simulink model "adaptive_control"  (R2020b)
settings: Solver=VariableStepAuto  StartTime=0.0  StopTime=30  RelTol=1e-3
values from neighbouring files (symbols this model uses):
  A = 1    [hw8_main.m]
  ddq_d = 0    [hw8_main.m]
  dq_d = 0    [hw8_main.m]
  F_hat0 = oneDof.F*0.8    [hw8_main.m]
  Fc = 1    [hw8_main.m]
  G_hat0 = oneDof.G*0.8    [hw8_main.m]
  I_hat0 = oneDof.I*0.8    [hw8_main.m]
  K_D = 100    [hw8_main.m]
  K_theta_inv = inv(K_theta)    [hw8_main.m]
  Lamba = 50    [hw8_main.m]
undefined symbols (not defined in the file or in its folder): oneDof
settings Model: Creator=nicol  LastModifiedBy=nicol

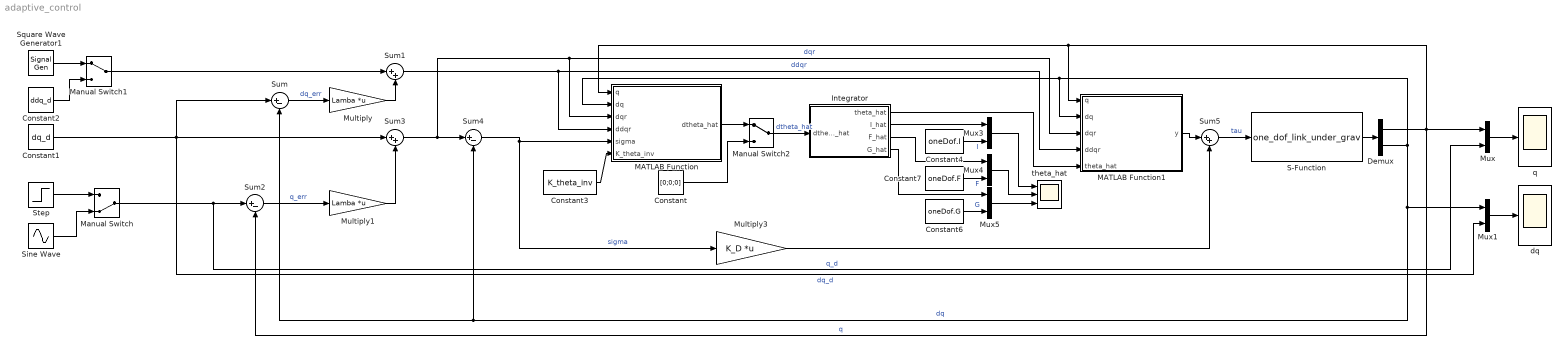
== system adaptive_control ==
  Constant : Constant  Value=[0;0;0]
  Constant1 : Constant  Value=dq_d
  Constant2 : Constant  Value=ddq_d
  Constant3 : Constant  Value=K_theta_inv
  Constant4 : Constant  Value=oneDof.I
  Constant6 : Constant  Value=oneDof.G
  Constant7 : Constant  Value=oneDof.F
  Demux : Demux  Outputs=2
  Integrator : Subsystem
  MATLAB Function : MATLAB Function  TreatAsAtomicUnit=on
  MATLAB Function1 : MATLAB Function  TreatAsAtomicUnit=on
  Manual Switch : ManualSwitch  CurrentSetting=0
  Manual Switch1 : ManualSwitch
  Manual Switch2 : ManualSwitch
  Multiply : Gain  Gain=Lamba  Multiplication=Matrix(K*u)
  Multiply1 : Gain  Gain=Lamba  Multiplication=Matrix(K*u)
  Multiply3 : Gain  Gain=K_D  Multiplication=Matrix(K*u)
  Mux{,1,3..5} (5 alike) : Mux  Inputs=2
  S-Function : S-Function  FunctionName=one_dof_link_under_grav  Parameters=oneDof  SFunctionDeploymentMode=off  EnableBusSupport=off
  Sine Wave : Sin  Amplitude=A  Frequency=Fc  SampleTime=0
  Square Wave Generator1 : SignalGenerator  WaveForm=square  Amplitude=A  Units=rad/sec
  Step : Step  After=A  SampleTime=0
  Sum : Sum  Inputs=|+-
  Sum1 : Sum  Inputs=|++
  Sum2 : Sum  Inputs=|+-
  Sum3 : Sum  Inputs=|++
  Sum4 : Sum  Inputs=|+-
  Sum5 : Sum  Inputs=|++
  dq : Scope
  q : Scope
  theta_hat : Scope  NumInputPorts=3
  wires:
  Sum/1 -> Multiply/1  "dq_err"
  Constant1/1 -> Mux1/2, Sum3/1, Sum/1  "dq_d"
  Manual Switch1/1 -> Sum1/1
  Multiply/1 -> Sum1/2
  Manual Switch/1 -> Mux/2, Sum2/1  "q_d"
  Sum2/1 -> Multiply1/1  "q_err"
  Sum3/1 -> Sum4/1, MATLAB Function/3(dqr), MATLAB Function1/3(dqr)  "dqr"
  Multiply1/1 -> Sum3/2
  Sum4/1 -> MATLAB Function/5(sigma), Multiply3/1  "sigma"
  MATLAB Function/1(dtheta_hat) -> Manual Switch2/1
  MATLAB Function1/1(y) -> Sum5/1
  Multiply3/1 -> Sum5/2
  Demux/1 -> MATLAB Function1/1(q), MATLAB Function/1(q), Mux/1, Sum2/2  "q"
  S-Function/1 -> Demux/1
  Sum5/1 -> S-Function/1  "tau"
  Demux/2 -> MATLAB Function1/2(dq), MATLAB Function/2(dq), Mux1/1, Sum4/2, Sum/2  "dq"
  Sum1/1 -> MATLAB Function/4(ddqr), MATLAB Function1/4(ddqr)  "ddqr"
  Mux1/1 -> dq/1
  Mux/1 -> q/1
  Constant3/1 -> MATLAB Function/6(K_theta_inv)
  Sine Wave/1 -> Manual Switch/2
  Square Wave Generator1/1 -> Manual Switch1/1
  Constant2/1 -> Manual Switch1/2
  Step/1 -> Manual Switch/1
  Constant/1 -> Manual Switch2/2
  Constant4/1 -> Mux3/2  "I"
  Mux4/1 -> theta_hat/2
  Constant7/1 -> Mux4/2  "F"
  Constant6/1 -> Mux5/2  "G"
  Mux5/1 -> theta_hat/3
  Mux3/1 -> theta_hat/1
  Manual Switch2/1 -> Integrator/1(dtheta_hat)  "dtheta_hat"
  Integrator/2(I_hat) -> Mux3/1
  Integrator/1(theta_hat) -> MATLAB Function1/5(theta_hat)
  Integrator/3(F_hat) -> Mux4/1
  Integrator/4(G_hat) -> Mux5/1

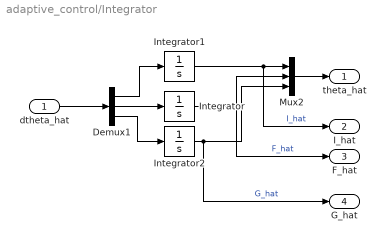
== system adaptive_control/Integrator ==
  dtheta_hat : Inport
  Demux1 : Demux  Outputs=3
  Integrator : Integrator  InitialCondition=F_hat0
  Integrator1 : Integrator  InitialCondition=I_hat0
  Integrator2 : Integrator  InitialCondition=G_hat0
  Mux2 : Mux  Inputs=3
  theta_hat : Outport
  I_hat : Outport  Port=2
  F_hat : Outport  Port=3
  G_hat : Outport  Port=4
  wires:
  Integrator/1 -> F_hat/1, Mux2/2  "F_hat"
  Mux2/1 -> theta_hat/1
  Demux1/2 -> Integrator/1
  Integrator1/1 -> I_hat/1, Mux2/1  "I_hat"
  Integrator2/1 -> G_hat/1, Mux2/3  "G_hat"
  dtheta_hat/1 -> Demux1/1
  Demux1/1 -> Integrator1/1
  Demux1/3 -> Integrator2/1

== matlab function adaptive_control/MATLAB Function1 ==
  data: q input; dq input; dqr input; ddqr input; theta_hat input; y output
function y = Y(q,dq,dqr,ddqr,theta_hat)
    Y=[ddqr dqr sin(q)];
y = Y*theta_hat;

== matlab function adaptive_control/MATLAB Function ==
  data: q input; dq input; dqr input; ddqr input; sigma input; dtheta_hat output; K_theta_inv input
function dtheta_hat = Y_transpose(q,dq,dqr,ddqr,sigma,K_theta_inv)
    Y=[ddqr dqr sin(q)];
dtheta_hat = K_theta_inv*Y'*sigma;
